simulink model "State_Transition_Table"  (R2025b)
settings: Solver=FixedStepDiscrete  StartTime=0.0  StopTime=10.0  FixedStep=0.01  RelTol=1e-3
libraries: simulink x1
settings Model: Creator=soura  LastModifiedBy=soura

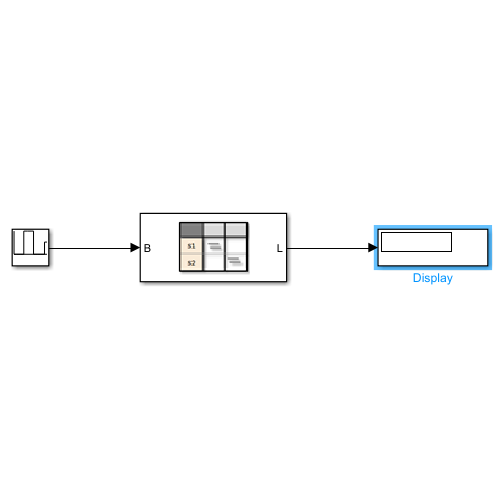
[thumbnail: Simulink's stored preview of the top-level diagram]
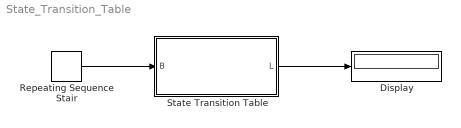
== system State_Transition_Table ==
  Display : Display
  Repeating Sequence Stair : simulink/Sources/Repeating Sequence Stair  OutValues=[0 0 0 1 1 1 0 0 0 0.5].'  tsamp=-1  OutMin=[]  OutMax=[]  OutDataTypeStr=double  OutputDataTypeScalingMode=double  OutDataType=fixdt(0,8)  ConRadixGroup=Best Precision: Vector-wise  OutScaling=2^-12
  State Transition Table : State Transition Table  TreatAsAtomicUnit=on
  wires:
  Repeating Sequence Stair/1 -> State Transition Table/1(B)
  State Transition Table/1(L) -> Display/1

== stateflow chart State_Transition_Table/State Transition Table ==
  state Off
  state On
  state Invalid
  (default) -> Off
  Off -> (junction 35) [order 2] : [B>0 && B<1]
  (junction 35) -> (junction 33)
  Off -> On [order 1] : [B==1]
      | {L=0}
  On -> Off [order 1] : [B==0]
      | {L=1}
  On -> Invalid [order 2] : [B>0 && B<1]
  Invalid -> (junction 37)
  (junction 37) -> Invalid
  (junction 33) -> Invalid
  data: L output; B input
